simulink model "v2_q_Control_PI"  (R2026a)
settings: Solver=FixedStepAuto  StopTime=inf  FixedStep=0.01  EnableMultiTasking=on
undefined symbols (not defined in the file or in its folder): Continuous, Time
libraries: arduinolib x3, simulink x1, arduinosensorlib x1, ctrlSharedLib x1, slpidlib x1
settings Model: SILPILModeSetting=veronly  ExtModeTrigDuration=2  Creator=Lenovo  LastModifiedBy=Lenovo
settings HardwareCC: ProdLargestAtomicInteger=Long  ProdLargestAtomicFloat=Double  ProdHWDeviceType=ARM Compatible->ARM Cortex
settings RTWCC: SystemTargetFile=ert.tlc  HardwareBoard=ESP32-WROOM (Arduino Compatible)  TLCOptions="-aInlineSetEventsForThisBaseRateFcn=TLC_FALSE -aSuppressMultiTaskScheduler=TLC_FALSE  -aRateBasedStepFcn=0"  Toolchain=ESP32  BuildConfiguration=Faster Runs  Description=Embedded Coder
settings ERTTargetCC: ExtModeTransport=3.0  ExtModeAutomaticAllocSize=off  ExtModeStaticAllocSize=65536.0  RootIOFormat=Structure reference  SupportContinuousTime=on  SupportVariableSizeSignals=on

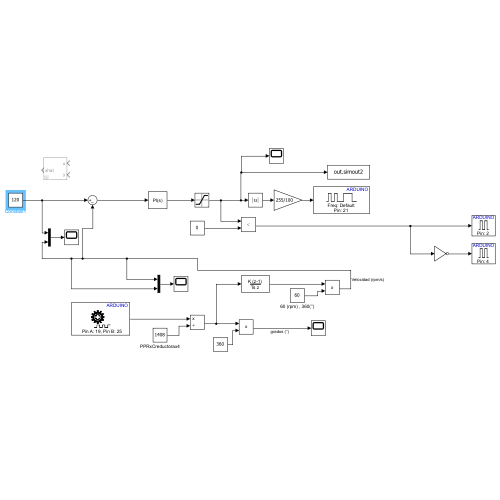
[thumbnail: Simulink's stored preview of the top-level diagram]
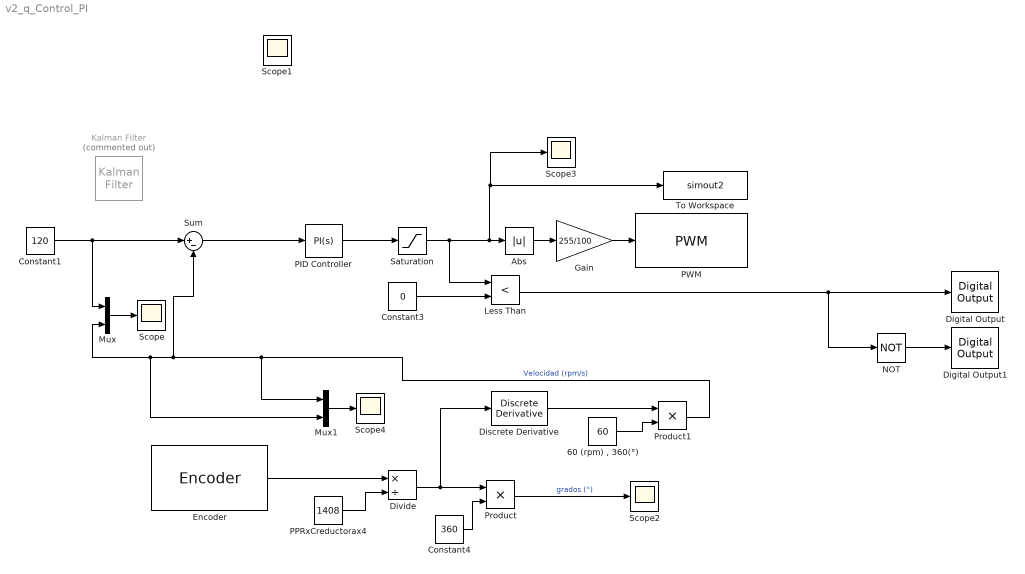
== system v2_q_Control_PI ==
  "60 (rpm) , 360(°)" : Constant  Value=60
  Abs : Abs  SaturateOnIntegerOverflow=off
  Constant1 : Constant  Value=120
  Constant3 : Constant  Value=0
  Constant4 : Constant  Value=360
  Digital Output : arduinolib/Digital Output  pinNumber=2  Direction=output  blockPlatform=arduino
  Digital Output1 : arduinolib/Digital Output  pinNumber=4  Direction=output  blockPlatform=arduino
  Discrete Derivative : simulink/Discrete/Discrete Derivative  gainval=1.0  ICPrevScaledInput=0.0  OutMin=[]  OutMax=[]  OutDataType=fixdt(1, 16)  OutScaling=2^-10  DoSatur=off
  Divide : Product  Inputs=*/
  Encoder : arduinosensorlib/Encoder  InputA=19  InputB=25  Mode=No reset  SampleTime=-1
  Gain : Gain  Gain=255/100
  Kalman Filter : ctrlSharedLib/Kalman Filter  Commented=on  TimeDomain=Continuous-Time  UseCurrentEstimator=on  ModelSource=Individual A, B, C, D matrices  ModelSourceVariable=Sd  A=-13.46  B=26.07  C=1  D=0  NumberOfStates=1  NumberOfInputs=1  NumberOfOutputs=1  Ts=-1  InitialEstimateSource=Dialog  X0=0  P0=10  UseK=off  UseGH=off  G=1  TimeInvariantG=on  H=0  TimeInvariantH=on  NumberOfProcessNoiseInputs=1  Q=0.1  TimeInvariantQ=on  R=0.1  TimeInvariantR=on  N=0  TimeInvariantN=on  AddInputPort=on  AddEnablePort=off  OutputEstimatedY=off  OutputP=off
  Less Than : RelationalOperator  Operator=<  OutDataTypeStr=boolean  RndMeth=Simplest  InputSameDT=off
  Mux : Mux  Inputs=2
  Mux1 : Mux  Inputs=2
  NOT : Logic  Operator=NOT  IconShape=distinctive  AllPortsSameDT=off  OutDataTypeStr=boolean
  PID Controller : slpidlib/PID Controller  Controller=PI  Form=Parallel  TimeDomain=Continuous-time  UseExternalTs=off  SampleTime=-1  IntegratorMethod=Forward Euler  FilterMethod=Forward Euler  ControllerParametersSource=internal  P=1.16905686651183  I=37.5967315261707  UseKiTs=off  D=0.286828849874282  UseExternalDerivativeSource=off  N=966.315735442536  UseFilter=on  TunerSelectOption=Transfer Function Based (PID Tuner App)  InitialConditionSource=internal  InitialConditionForIntegrator=0  InitialConditionForFilter=0  DifferentiatorICPrevScaledInput=0  ExternalReset=none  TrackingMode=off  Kt=1  LimitOutput=off  SatLimitsSource=internal  UpperSaturationLimit=inf  LowerSaturationLimit=-inf  LinearizeAsGain=on  AntiWindupMode=none  Kb=1  LimitIntegrator=off  UpperIntegratorSaturationLimit=inf  LowerIntegratorSaturationLimit=-inf  POutMin=[]  POutMax=[]  IOutMin=[]  IOutMax=[]  DOutMin=[]  DOutMax=[]  NOutMin=[]  NOutMax=[]  SumOutMin=[]  SumOutMax=[]  SaturationOutMin=[]  SaturationOutMax=[]  PParamMin=[]  PParamMax=[]  IParamMin=[]  IParamMax=[]  DParamMin=[]  DParamMax=[]  NParamMin=[]  NParamMax=[]  KbParamMin=[]  KbParamMax=[]  KtParamMin=[]  KtParamMax=[]  KbOutMin=[]  KbOutMax=[]  KtOutMin=[]  KtOutMax=[]  IntegratorOutMin=[]  IntegratorOutMax=[]  FilterOutMin=[]  FilterOutMax=[]  SumI1OutMin=[]  SumI1OutMax=[]  SumI2OutMin=[]  SumI2OutMax=[]  SumI3OutMin=[]  SumI3OutMax=[]  SumI4OutMin=[]  SumI4OutMax=[]  SumDOutMin=[]  SumDOutMax=[]  DifferentiatorOutMin=[]  DifferentiatorOutMax=[]  FilterDiffOutCoefMin=[]  FilterDiffOutCoefMax=[]  ReciprocalOutMin=[]  ReciprocalOutMax=[]  SumDenOutMin=[]  SumDenOutMax=[]  SumNumOutMin=[]  SumNumOutMax=[]  DivideOutMin=[]  DivideOutMax=[]  UdiffTsProdOutMin=[]  UdiffTsProdOutMax=[]  NTsProdOutMin=[]  NTsProdOutMax=[]  UintegralTsProdOutMin=[]  UintegralTsProdOutMax=[]  UngainTsProdOutMin=[]  UngainTsProdOutMax=[]  ClampingZeroOutDataTypeStr=Inherit: Inherit via back propagation  ClampingZeroOutMin=[]  ClampingZeroOutMax=[]  FilterDenConstantOutDataTypeStr=Inherit: Inherit via back propagation  FilterDenConstantOutMin=[]  FilterDenConstantOutMax=[]  PCopyOutDataTypeStr=Inherit: Inherit via back propagation  PCopyOutMin=[]  PCopyOutMax=[]  NCopyOutDataTypeStr=Inherit: Inherit via back propagation  NCopyOutMin=[]  NCopyOutMax=[]  IntegratorContinuousStateAttributes=''  IntegratorStateMustResolveToSignalObject=off  IntegratorRTWStateStorageClass=Auto  FilterContinuousStateAttributes=''  FilterStateMustResolveToSignalObject=off  FilterRTWStateStorageClass=Auto  ParallelPVariant=InternalParameters  IdealPVariant=Disabled  IVariant=InternalParameters  DVariant=Disabled  IntegratorVariant=Continuous  SatVariant=Disabled  AWVariant=Passthrough  PCopyVariant=Disabled  TRVariant=Disabled  FdbkBlocksVariant=Forward  IdealPFdbkVariant=Disabled  SatFdbkVariant=Disabled  DerivativeFilterVariant=Disabled  NVariant=Disabled  NCopyVariant=Disabled_SignalSpec  FilterICVariant=Disabled  IntegratorICVariant=InternalICs  ExternalResetVariant=Disabled  TRSumVariant=Passthrough  SumFdbkVariant=Disabled  SumVariant=Sum_PI  TsampFilterVariant=InternalTs  TsampNgainVariant=Passthrough  TsampIntegralVariant=Disabled_SignalSpec  ExternalSaturationOutDataTypeStr=Inherit: Same as second input  DerivativeSourceVariant=Disabled  PreIntVariant=InternalPreInt
  PPRxCreductorax4 : Constant  Value=1408
  PWM : arduinolib/PWM  pinNumber=21  frequencyType=Default  desiredFrequency=490.2  achievableFrequency=490.2
  Product : Product
  Product1 : Product
  Saturation : Saturate  UpperLimit=100  LowerLimit=-100
  Scope{,1..4} (5 alike) : Scope
      Scope settings: ActiveDisplayYMinimum=41.015624999986358  ActiveDisplayYMaximum=142.22301136363512
      Scope2 settings: ActiveDisplayYMinimum=-5504.7975852272721  ActiveDisplayYMaximum=49543.178267045456  DataLoggingVariableName=ScopeData2
      Scope3 settings: ActiveDisplayYMinimum=-125  ActiveDisplayYMaximum=125  DataLoggingVariableName=ScopeData3
      Scope4 settings: ActiveDisplayYMinimum=2.8315898357625642  ActiveDisplayYMaximum=94.143516767661453  DataLoggingVariableName=ScopeData4
  Sum : Sum  Inputs=|+-
  To Workspace : ToWorkspace  VariableName=simout2  SaveFormat=Structure With Time  SampleTime=-1
  wires:
  Encoder/1 -> Divide/1
  PPRxCreductorax4/1 -> Divide/2
  Divide/1 -> Discrete Derivative/1, Product/1
  Constant4/1 -> Product/2
  Product/1 -> Scope2/1  "grados (°)"
  Discrete Derivative/1 -> Product1/1
  "60 (rpm) , 360(°)"/1 -> Product1/2
  Product1/1 -> Sum/2, Mux1/2, Mux/2, Mux1/1  "Velocidad (rpm/s)"
  Gain/1 -> PWM/1
  Constant1/1 -> Mux/1, Sum/1
  Mux/1 -> Scope/1
  Sum/1 -> PID Controller/1
  PID Controller/1 -> Saturation/1
  Abs/1 -> Gain/1
  Saturation/1 -> Less Than/1, Scope3/1, To Workspace/1, Abs/1
  Constant3/1 -> Less Than/2
  Less Than/1 -> NOT/1, Digital Output/1
  NOT/1 -> Digital Output1/1
  Mux1/1 -> Scope4/1
